simulink model "mInterpolatedStateSpaceThermalModel_OneCoolSys"  (R2021b)
settings: Solver=VariableStepAuto  StartTime=0.0  StopTime=4000  FixedStep=0.2  RelTol=1e-3  AbsTol=1e-3
values from neighbouring files (symbols this model uses):
  TnodesInit = [TcoolantIn;330;290]    [tInterpolatedStateSpaceThermalModel.m]
libraries: mcadROM_lib x1
settings Model: Creator=agonzale  LastModifiedBy=agonzale
settings SolverCC: AutoScaleAbsTol=off  NumberNewtonIterations=3

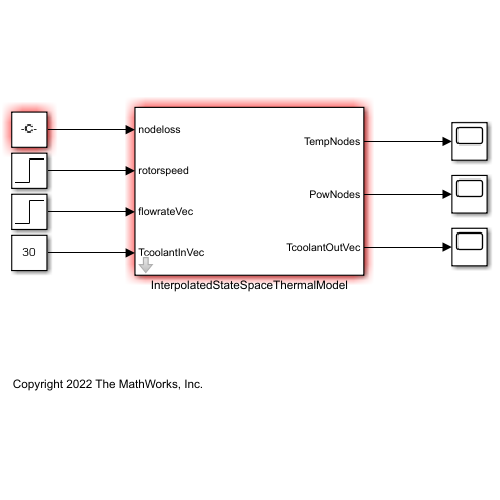
[thumbnail: Simulink's stored preview of the top-level diagram]
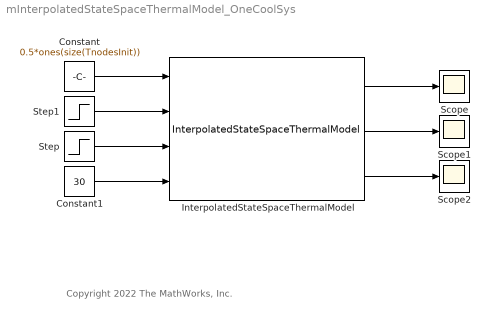
== system mInterpolatedStateSpaceThermalModel_OneCoolSys ==
  note: Copyright 2022 The MathWorks, Inc.
  Constant : Constant  Value=0.5*ones(size(TnodesInit))
  Constant1 : Constant  Value=30
  InterpolatedStateSpaceThermalModel : mcadROM_lib/InterpolatedStateSpaceThermalModel  BkptsStruct=BkptsStruct  AMatND=AmatND  BMatND=BmatND  ResMatND=ResMatND  CoolAdjMat=AdjacencyMat  CoolantArrayIdxs=[5 25] % dummy value  InletCoolantIdxs=InletCoolIdxs  OutletCoolantIdxs=OutletCoolIdxs  TnodesInit=TnodesInit
  Scope : Scope
  Scope1 : Scope
  Scope2 : Scope
  Step : Step  Time=1000  Before=5  After=9  SampleTime=0
  Step1 : Step  Time=500  Before=1000  After=3000  SampleTime=0
  wires:
  Constant/1 -> InterpolatedStateSpaceThermalModel/1
  Step1/1 -> InterpolatedStateSpaceThermalModel/2
  Step/1 -> InterpolatedStateSpaceThermalModel/3
  Constant1/1 -> InterpolatedStateSpaceThermalModel/4
  InterpolatedStateSpaceThermalModel/1 -> Scope/1
  InterpolatedStateSpaceThermalModel/2 -> Scope1/1
  InterpolatedStateSpaceThermalModel/3 -> Scope2/1
